simulink model "Stop_Generated"  (R2019a)
settings: Solver=ode3  StartTime=0.0  StopTime=inf  FixedStep=0.1  RelTol=1e-3  EnableMultiTasking=on
libraries: simulink x1
settings Model: Creator=david  LastModifiedBy=david
settings DataIOCC: LimitDataPoints=on  SaveFormat=Array  ReturnWorkspaceOutputs=off
settings OptimizationCC: DefaultParameterBehavior=Inlined  InlineInvariantSignals=on  PassReuseOutputArgsAs=Individual arguments  LifeSpan=inf
settings DebuggingCC: ParameterTunabilityLossMsg=error
settings HardwareCC: ProdBitPerPointer=32  ProdBitPerSizeT=32  ProdBitPerPtrDiffT=32  ProdLargestAtomicFloat=None  ProdWordSize=32  ProdHWDeviceType=Custom Processor->Custom Processor
settings ModelReferenceCC: PropagateSignalLabelsOutOfModel=off
settings SFSimCC: MATLABDynamicMemAlloc=off
settings RTWCC: SystemTargetFile=ert.tlc  GenCodeOnly=on  TemplateMakefile=ert_default_tmf  IncludeHyperlinkInReport=on
settings CodeAppCC: IgnoreCustomStorageClasses=off  StateflowObjectComments=on
settings ERTTargetCC: IncludeMdlTerminateFcn=off  SupportAbsoluteTime=off  MultiInstanceERTCode=on  CodeInterfacePackaging=Reusable function  PurelyIntegerCode=on  SupportNonFinite=off  SupportComplex=off  InlinedParameterPlacement=NonHierarchical  MultiInstanceErrorCode=None  ERTCustomFileTemplate=example_file_process.tlc  ConvertIfToSwitch=off  SuppressUnreachableDefaultCases=off

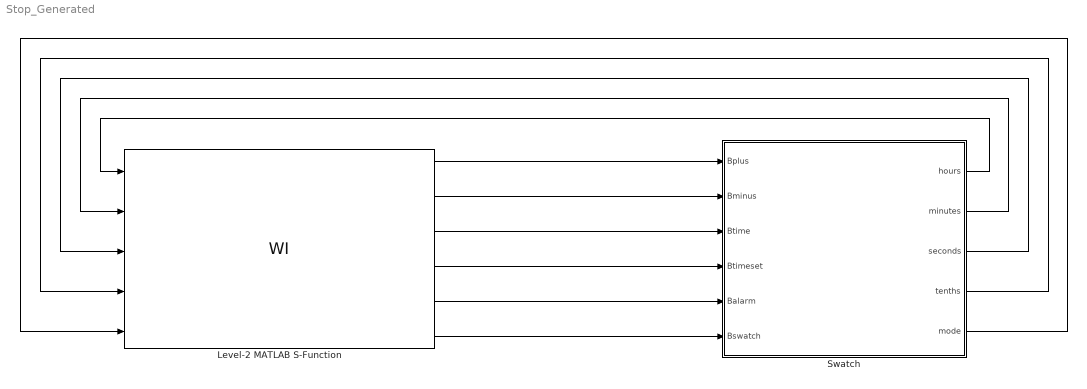
== system Stop_Generated ==
  Level-2 MATLAB S-Function : M-S-Function  FunctionName=WI
  "Swatch  " : Subsystem
  wires:
  Level-2 MATLAB S-Function/1 -> "Swatch  "/1(Bplus)
  Level-2 MATLAB S-Function/2 -> "Swatch  "/2(Bminus)
  Level-2 MATLAB S-Function/3 -> "Swatch  "/3(Btime)
  Level-2 MATLAB S-Function/4 -> "Swatch  "/4("Btimeset ")
  Level-2 MATLAB S-Function/5 -> "Swatch  "/5(Balarm)
  Level-2 MATLAB S-Function/6 -> "Swatch  "/6(Bswatch)
  "Swatch  "/1(hours) -> Level-2 MATLAB S-Function/1
  "Swatch  "/2(minutes) -> Level-2 MATLAB S-Function/2
  "Swatch  "/3(seconds) -> Level-2 MATLAB S-Function/3
  "Swatch  "/4(tenths) -> Level-2 MATLAB S-Function/4
  "Swatch  "/5(mode) -> Level-2 MATLAB S-Function/5

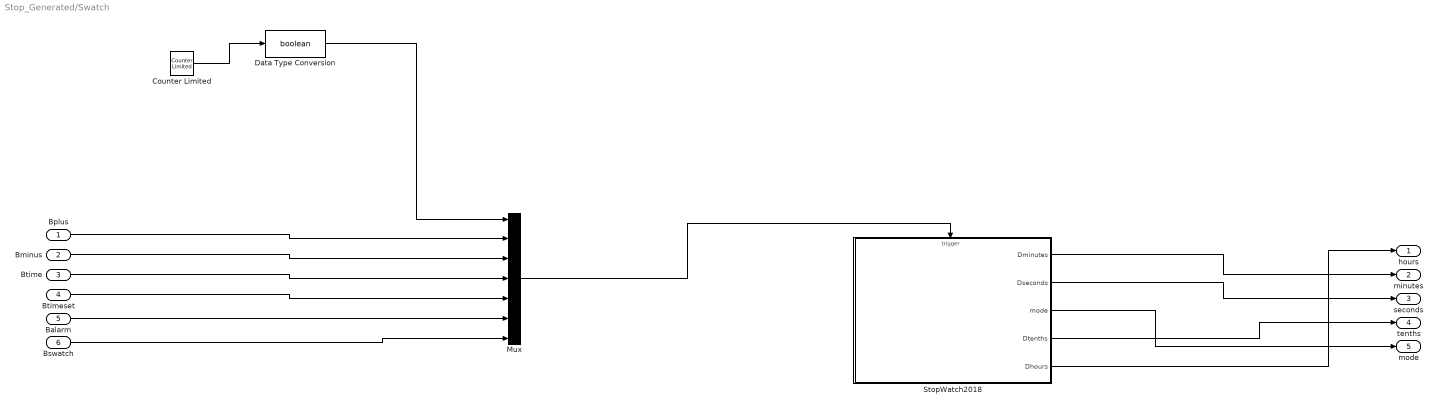
== system Stop_Generated/Swatch   ==
  Bplus : Inport
  Bminus : Inport  Port=2
  Btime : Inport  Port=3
  "Btimeset " : Inport  Port=4
  Balarm : Inport  Port=5
  Bswatch : Inport  Port=6
  Counter Limited : simulink/Sources/Counter Limited  uplimit=1  tsamp=0.1
  Data Type Conversion : DataTypeConversion  OutDataTypeStr=boolean
  Mux : Mux  Inputs=7
  "StopWatch2018 " : Stateflow chart  BlockKeywords=__PRM__SERIALIZED__DATA__:Stateflow Chart,Stateflow Diagram  TreatAsAtomicUnit=on
  hours : Outport
  minutes : Outport  Port=2
  seconds : Outport  Port=3
  tenths : Outport  Port=4
  mode : Outport  Port=5
  wires:
  Bplus/1 -> Mux/2
  Bminus/1 -> Mux/3
  Data Type Conversion/1 -> Mux/1
  Btime/1 -> Mux/4
  "Btimeset "/1 -> Mux/5
  Mux/1 -> "StopWatch2018 "/Trigger
  Counter Limited/1 -> Data Type Conversion/1
  Bswatch/1 -> Mux/7
  Balarm/1 -> Mux/6
  "StopWatch2018 "/3(mode) -> mode/1
  "StopWatch2018 "/4(Dtenths) -> tenths/1
  "StopWatch2018 "/2(Dseconds) -> seconds/1
  "StopWatch2018 "/1(Dminutes) -> minutes/1
  "StopWatch2018 "/5(Dhours) -> hours/1

== stateflow chart Stop_Generated/Swatch  /StopWatch2018  ==
  state AlarmManagement [parallel]
    settings: executionOrder=1
    state Checking
    state Buzzer_ON
    (default) -> Checking
    Checking -> Buzzer_ON : [Ahours == hours && Aminutes == minutes]
    Buzzer_ON -> Checking : [Ahours ~= hours || Aminutes ~= minutes]
  state TimeCount [parallel]
    settings: executionOrder=2
    state Count
    (junction 61) -> Count
    (default) -> Count : {Dtenths = uint8(0);
        | tenths = uint8(0);}
    (junction 52) -> Count [order 1] : {hours = hours +1}
    (junction 51) -> Count [order 2] : {minutes = minutes +1;}
    (junction 50) -> Count [order 2] : {seconds = seconds + 1;}
    Count -> (junction 49) : Tick
    (junction 49) -> (junction 50) [order 1] : [tenths == 9]{tenths = uint8(0);}
    (junction 50) -> (junction 51) [order 1] : [seconds == 59]{seconds = uint8(0);}
    (junction 51) -> (junction 52) [order 1] : [minutes == 59]{minutes = uint8(0);}
    (junction 52) -> (junction 61) [order 2] : [hours == 24]{hours = uint8(0)}
    (junction 49) -> Count [order 2] : {tenths = tenths +1;}
    TimeCount -> Count : StopW_Start
  state TimeCountStopWatch [parallel]
    settings: executionOrder=3
    state Stop_WithOut_Update
    state S_Count
    S_Count -> Stop_WithOut_Update [order 2] : plusbutton
    (junction 194) -> S_Count
    (default) -> S_Count
    (junction 180) -> S_Count [order 2] : {Shours = hours +1}
    (junction 187) -> S_Count [order 2] : {Sminutes = Sminutes +1;}
    (junction 192) -> S_Count [order 2] : {Sseconds = Sseconds + 1;}
    (junction 192) -> (junction 187) [order 1] : [Sseconds == 59]{Sseconds = uint8(0);}
    (junction 187) -> (junction 180) [order 1] : [Sminutes == 59]{Sminutes = uint8(0);}
    (junction 180) -> (junction 194) [order 1] : [Shours == 24]{Shours = uint8(0)}
    (junction 179) -> (junction 192) [order 1] : [Stenths == 9]{Stenths = uint8(0);}
    (junction 179) -> S_Count [order 2] : {Stenths = Stenths +1;}
    S_Count -> (junction 179) [order 1] : Tick
    TimeCountStopWatch -> S_Count : StopW_Start
  state interface [parallel]
    settings: executionOrder=4
    state TimeDisplay
      en: mode = uint8(0)
      du: Dhours = hours;
      Dminutes = minutes;
      Dtenths = tenths;
      Dseconds = seconds
    state TimeSetting
      en: mode = uint8(1)
      state Set_H
        Dhours = hours;
      state Set_M
        Dminutes = minutes
      interface.TimeSetting.Set_H -> (junction 164) [order 2] : plusbutton
      (junction 164) -> interface.TimeSetting.Set_H [order 1] : [hours < 23]{hours = hours +1;}
      (junction 164) -> interface.TimeSetting.Set_H [order 2] : [hours == 23]{hours = uint8(0);}
      (junction 174) -> interface.TimeSetting.Set_M [order 2] : {minutes = minutes +1;}
      (default) -> interface.TimeSetting.Set_H
      (junction 174) -> interface.TimeSetting.Set_M [order 1] : [minutes == 59]{minutes = uint8(0);}
      interface.TimeSetting.Set_M -> (junction 174) [order 1] : plusbutton
      interface.TimeSetting.Set_H -> interface.TimeSetting.Set_M [order 1] : timesetmode
      interface.TimeSetting.Set_M -> interface.TimeSetting.Set_H [order 3] : timesetmode
      (junction 160) -> interface.TimeSetting.Set_H [order 1] : [hours ==0]{hours = 23;}
      (junction 156) -> interface.TimeSetting.Set_M [order 2] : {minutes = minutes -1;}
      interface.TimeSetting.Set_M -> (junction 156) [order 2] : minusbutton
      (junction 156) -> interface.TimeSetting.Set_M [order 1] : [minutes ==0]{minutes = 59;}
      (junction 160) -> interface.TimeSetting.Set_H [order 2] : {hours = hours -1;}
      interface.TimeSetting.Set_H -> (junction 160) [order 3] : minusbutton
    state Alarm
      en: mode = uint8(2)
      state Set_M
        Dminutes = Aminutes
      state Set_H
        Dhours = Ahours;
      interface.Alarm.Set_H -> (junction 139) [order 1] : plusbutton
      (junction 139) -> interface.Alarm.Set_H [order 1] : [Ahours < 23]{Ahours = Ahours +1;}
      (junction 139) -> interface.Alarm.Set_H [order 2] : [Ahours == 23]{Ahours = uint8(0);}
      (junction 147) -> interface.Alarm.Set_M [order 2] : {Aminutes = Aminutes +1;}
      interface.Alarm.Set_M -> (junction 147) [order 1] : plusbutton
      (junction 147) -> interface.Alarm.Set_M [order 1] : [Aminutes == 59]{Aminutes = uint8(0);}
      (default) -> interface.Alarm.Set_H
      interface.Alarm.Set_H -> interface.Alarm.Set_M [order 3] : alarmmode
      interface.Alarm.Set_M -> interface.Alarm.Set_H [order 3] : alarmmode
      (junction 151) -> interface.Alarm.Set_M [order 2] : {Aminutes = Aminutes -1;}
      interface.Alarm.Set_M -> (junction 151) [order 2] : minusbutton
      (junction 151) -> interface.Alarm.Set_M [order 1] : [Aminutes ==0]{Aminutes = 59;}
      (junction 144) -> interface.Alarm.Set_H [order 1] : [Ahours ==0]{Ahours = 23;}
      (junction 144) -> interface.Alarm.Set_H [order 2] : {Ahours = Ahours -1;}
      interface.Alarm.Set_H -> (junction 144) [order 2] : minusbutton
    state StopWatch
      en: mode = uint8(3);
      Shours = uint8(0);
      Sminutes = uint8(0);
      Sseconds = uint8(0);
      Stenths = uint8(0);
      Dhours = uint8(0);
      Dminutes =uint8(0);
      Dseconds = uint8(0);
      Dtenths = uint8(0)
      state S_Start
        Dhours = Shours;
        Dminutes =Sminutes;
        Dseconds = Sseconds;
        Dtenths = Stenths
      state Wait_SWatch
      state S_Pause_With_Update
      (default) -> Wait_SWatch
      Wait_SWatch -> S_Start [order 1] : plusbutton{StopW_Start}
      S_Start -> Wait_SWatch [order 1] : plusbutton{StopW_Stop}
      Wait_SWatch -> Wait_SWatch [order 2] : swatchmode{
          | Shours = uint8(0);
          |  Sminutes = uint8(0);
          |  Sseconds = uint8(0);
          |  Stenths = uint8(0);
          | Dhours = uint8(0);
          | Dminutes =uint8(0);
          | Dseconds = uint8(0);
          | Dtenths = uint8(0)}
      S_Pause_With_Update -> S_Start : minusbutton
      S_Start -> S_Pause_With_Update [order 2] : minusbutton
    interface -> TimeDisplay [order 1] : timemode
    TimeDisplay -> TimeSetting [order 2] : timesetmode
    (default) -> TimeDisplay : {hours = uint8(1);
        | minutes = uint8(0);
        | seconds = uint8(45);
        | tenths = uint8(0);
        | Aminutes = uint8(1);
        | Ahours = uint8(1);
        | Shours = uint8(0);
        |  Sminutes = uint8(0);
        |  Sseconds = uint8(0);
        |  Stenths = uint8(0)}
    TimeDisplay -> Alarm [order 1] : alarmmode
    StopWatch -> Alarm [order 1] : alarmmode
    Alarm -> TimeSetting : timesetmode
    StopWatch -> TimeSetting [order 2] : timesetmode
    TimeSetting -> Alarm : alarmmode
    interface -> StopWatch [order 2] : swatchmode
  (default) -> interface
  data: Ahours local uint8; Aminutes local uint8; hours local uint8; seconds local uint8; tenths local uint8; Shours local uint8; Sminutes local uint8; Stenths local uint8; Sseconds local uint8; Dminutes output uint8; Dseconds output uint8; mode output uint8; Dtenths output uint8; Dhours output uint8; minutes local uint8
  events: Tick input RISING_EDGE_EVENT; StopW_Start local FUNCTION_CALL_EVENT; StopW_Stop local FUNCTION_CALL_EVENT; plusbutton input RISING_EDGE_EVENT; minusbutton input RISING_EDGE_EVENT; timemode input RISING_EDGE_EVENT; timesetmode input RISING_EDGE_EVENT; alarmmode input RISING_EDGE_EVENT; swatchmode input RISING_EDGE_EVENT
